simulink subsystem "ApplicationMotorSwap"  (R2023b)
settings: Solver=VariableStepAuto  StartTime=0.0  StopTime=10.0  RelTol=1e-3
values from neighbouring files (symbols this model uses):
  Ts_speed = 10*Ts    [mcbMotorSwapData.m]
settings Model: Creator=The MathWorks, Inc.  LastModifiedBy=snarayan

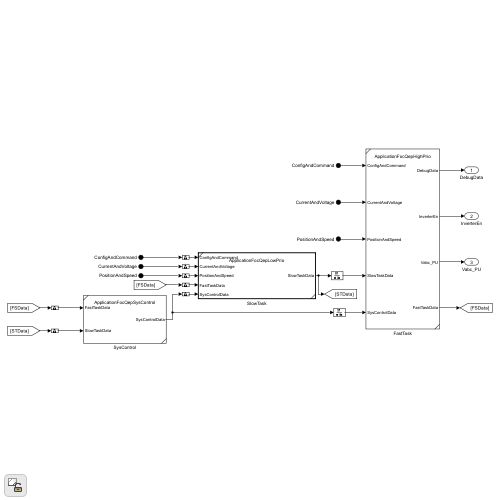
[thumbnail: Simulink's stored preview of the top-level diagram]
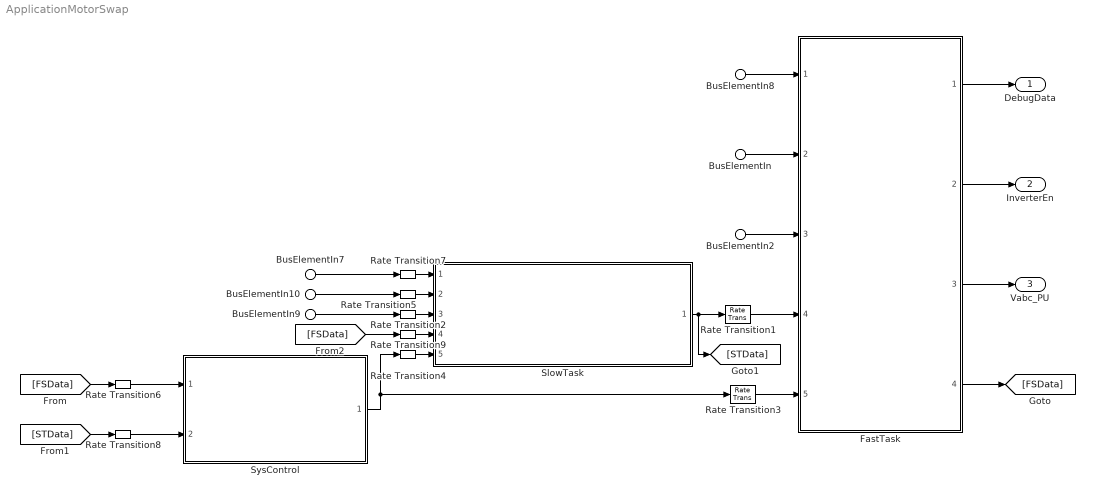
== system ApplicationMotorSwap ==
  BusElementIn7 : Inport  PortName=ConfigAndCommand
  BusElementIn8 : Inport  PortName=ConfigAndCommand
  BusElementIn10 : Inport  Port=2  PortName=CurrentAndVoltage
  BusElementIn : Inport  Port=2  PortName=CurrentAndVoltage
  BusElementIn9 : Inport  Port=3  PortName=PositionAndSpeed
  BusElementIn2 : Inport  Port=3  PortName=PositionAndSpeed
  FastTask : Subsystem  ReferencedSubsystem=ApplicationFocQepHighPrio
  Rate Transition1 : RateTransition  Deterministic=off  OutPortSampleTime=Ts
  Rate Transition{2,4..5,7,9} (5 alike) : RateTransition  Deterministic=off  OutPortSampleTime=Ts_speed
  Rate Transition3 : RateTransition  Deterministic=off  OutPortSampleTime=Ts
  Rate Transition6 : RateTransition  Deterministic=off  OutPortSampleTime=0.1
  Rate Transition8 : RateTransition  Deterministic=off  OutPortSampleTime=0.1
  SlowTask : Subsystem  TreatAsAtomicUnit=on  SystemSampleTime=Ts_speed  ReferencedSubsystem=ApplicationFocQepLowPrio
  SysControl : Subsystem  ReferencedSubsystem=ApplicationFocQepSysControl
  DebugData : Outport
  InverterEn : Outport  Port=2
  Vabc_PU : Outport  Port=3
  wires:
  FastTask/2 -> InverterEn/1
  FastTask/1 -> DebugData/1
  FastTask/3 -> Vabc_PU/1
  BusElementIn7/1 -> Rate Transition7/1
  Rate Transition7/1 -> SlowTask/1
  BusElementIn8/1 -> FastTask/1
  Rate Transition4/1 -> SlowTask/5
  SysControl/1 -> Rate Transition4/1, Rate Transition3/1
  BusElementIn9/1 -> Rate Transition2/1
  Rate Transition2/1 -> SlowTask/3
  BusElementIn10/1 -> Rate Transition5/1
  Rate Transition5/1 -> SlowTask/2
  BusElementIn/1 -> FastTask/2
  BusElementIn2/1 -> FastTask/3
  Rate Transition3/1 -> FastTask/5
  Rate Transition1/1 -> FastTask/4
  SlowTask/1 -> [STData], Rate Transition1/1
  FastTask/4 -> [FSData]
  Rate Transition6/1 -> SysControl/1
  [FSData] -> Rate Transition6/1
  [STData] -> Rate Transition8/1
  Rate Transition8/1 -> SysControl/2
  Rate Transition9/1 -> SlowTask/4
  [FSData] -> Rate Transition9/1
